simulink model "InvPendulum"  (R2018b)
settings: Solver=ode5  StartTime=0.0  StopTime=inf  FixedStep=0.01  RelTol=1e-3  AbsTol=1e-6
undefined symbols (not defined in the file): Standard_Devices, UDP_Protocol
libraries: sldrtlib x2, simulink x1
settings Model: ExtModeTrigDuration=18000  ExtModeTrigLevel=0.400000  Creator=jims  LastModifiedBy=Aleksei Tepljakov
settings SolverCC: AutoScaleAbsTol=off
settings DataIOCC: ExternalInput=[]  InitialState=[]  MaxDataPoints=5000  SaveFormat=Array  SignalLoggingSaveFormat=ModelDataLogs  SaveOutput=off  SaveTime=off
settings OptimizationCC: BooleanDataType=off  ExpressionDepthLimit=2147483647  LifeSpan=inf
settings DebuggingCC: SaveWithParameterizedLinksMsg=none  UnderspecifiedInitializationDetection=Classic  MergeDetectMultiDrivingBlocksExec=none  SignalResolutionControl=TryResolveAllWithWarning  MultiTaskDSMMsg=warning  MultiTaskCondExecSysMsg=none  IntegerOverflowMsg=none  FcnCallInpInsideContextMsg=warning  StateNameClashWarn=warning  SFUnexpectedBacktrackingDiag=warning  SFNoUnconditionalDefaultTransitionDiag=warning  SFExecutionAtInitializationDiag=none  IntegerSaturationMsg=none
settings HardwareCC: TargetBitPerLong=64  TargetBitPerPointer=64  TargetIntDivRoundTo=Zero  TargetEndianess=LittleEndian  TargetWordSize=64  TargetHWDeviceType=Intel->x86-64
settings ModelReferenceCC: PropagateSignalLabelsOutOfModel=off
settings SFSimCC: SimUseLocalCustomCode=off
settings RTWCC: SystemTargetFile=sldrt.tlc  TemplateMakefile=sldrt.tmf  Description=Simulink Desktop Real-Time  RTWUseLocalCustomCode=off  RTWCompilerOptimization=on
settings CodeAppCC: MaxIdLength=95  StateflowObjectComments=on
settings SimulinkDesktopRealTimeCC: TargetPreCompLibLocation=C:\Program Files\MATLAB\R2018b\toolbox\sldrt\lib\win64  TargetLangStandard=C89/C90 (ANSI)  SupportVariableSizeSignals=off  PreserveStateflowLocalDataDimensions=off
settings ConfigComp: CovMetricSettings=dw  CovHtmlReporting=on  CovSaveCumulativeToWorkspaceVar=on  CovSaveSingleToWorkspaceVar=on  CovExternalEMLEnable=off

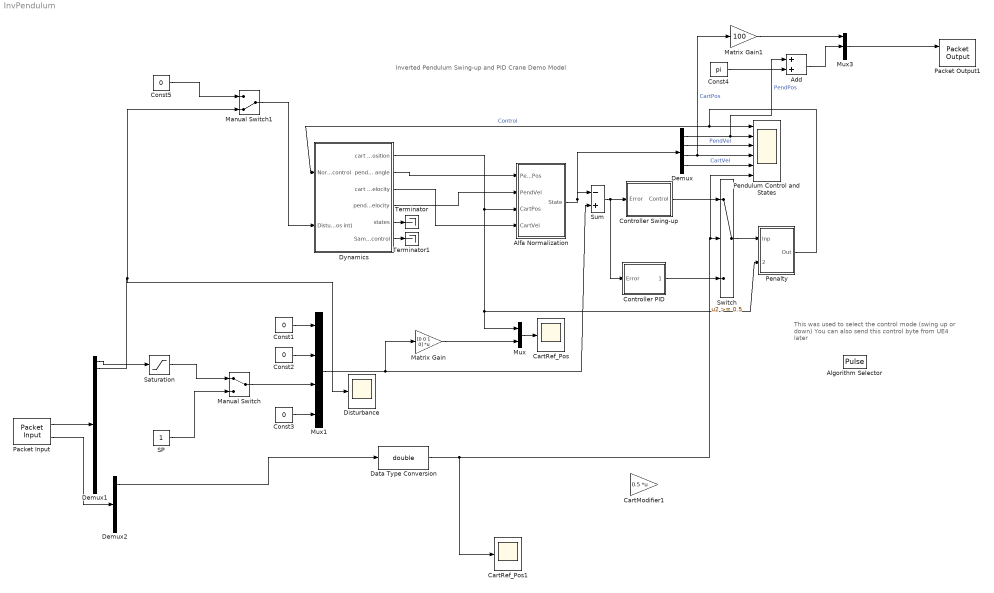
== system InvPendulum ==
  note: This was used to select
      | the control mode (swing up or down)
      | You can also send this control byte from UE4 later
  note: Inverted Pendulum
      | Swing-up and PID Crane Demo Model
  Add : Sum
  Alfa Normalization : Subsystem  mask(Choose mode:){}
  Algorithm Selector : DiscretePulseGenerator  PulseType=Time based  Period=30  PulseWidth=70
  CartModifier1 : Gain  Gain=0.5  Multiplication=Matrix(K*u)  SaturateOnIntegerOverflow=on  OutDataTypeStr=Inherit: Same as input  ParamDataTypeStr=Inherit: Same as input
  CartRef_Pos : Scope
  CartRef_Pos1 : Scope
  Const{1..3,5} (4 alike) : Constant  Value=0
  Const4 : Constant  Value=pi
  Controller PID : Subsystem  mask{Cart_PID=[ 0.5 0 0 ], Pend_PID=[ -1 0 -0.0 ], Umax=0.2, zone=1, Friction=0.03, T0=0.01}
      mask prompts: Cart_PID "Cart PID parameters [Kp, Ki, Kd]:"; Pend_PID "Pendulum PID parameters [Kp, Ki, Kd]:"; Umax "Maximum control value:"; zone "Stabilisation zone [rad]:"; Friction "Friction compensation:"; T0 "Sample time:"
  Controller Swing-up : Subsystem
  Data Type Conversion : DataTypeConversion  OutDataTypeStr=double
  Demux : Demux
  Demux1 : Demux  Outputs=20
  Demux2 : Demux  Outputs=3
  Disturbance : Scope
  Dynamics : Subsystem  mask(Dynamics){x_ini=[0, pi, 0, 0], m=[0.5723, 0.12], fr=[0.00027344,  1.1975875,  0.5], P4=[0.01955717, 0.0038583, 9.81], Up=[ 12.86, 0.093125], DZ=[0.1, 1.5]}
      mask prompts: x_ini "Initial state vector [x1(0)  x2(0)  x3(0)  x4(0)]"; m "mass of cart (mc)  mass of pendulum (mp)"; fr "friction :  fp  FS  FC"; P4 "Distance (l), Total Inertia moment (J), gravity (g)"; Up "control : magnitude (M)    DZu"; DZ "minimal velocities : cart (DZcv)  pendulum (DZcp)"
      mask help:
      | Pendulum-Cart Dynamics
      |
      | Copyright INTECO 1997
      mask init:
      | DZcv=DZ(1);DZcp=DZ(2);DZu=Up(2);l=P4(1);J=P4(2);g=P4(3);M=Up(1);mc=m(1);mp=m(2);fp=fr(1);FS=fr(2);FC=fr(3);mi=l*(mc+mp);a=l*l+J/(mc+mp);
      mask Display: plot(0,0,100,100,[40,48,48,40,40],[60,60,49,49,60],[37,44],[9,54],[100,8,4,1,0,100,100,0,40,100,100,0,0,40],[44,44,44,44,45,46,45,44,45,45,43,43,46,46],[100,48],[55,55],[0,40],[55,55])
  Manual Switch : ManualSwitch
  Manual Switch1 : ManualSwitch  CurrentSetting=0
  Matrix Gain : Gain  Gain=[0 0 1 0]  Multiplication=Matrix(K*u)  SaturateOnIntegerOverflow=on  OutDataTypeStr=Inherit: Same as input  ParamDataTypeStr=Inherit: Same as input
  Matrix Gain1 : Gain  Gain=100  SaturateOnIntegerOverflow=on  OutDataTypeStr=Inherit: Same as input  ParamDataTypeStr=Inherit: Same as input
  Mux : Mux  Inputs=2
  Mux1 : Mux
  Mux3 : Mux  Inputs=3
  Packet Input : sldrtlib/Packet Input  SampleTime=0.01  MaxMissedTicks=10  ShowMissedTicks=off  YieldWhenWaiting=off  DrvName=Standard_Devices/UDP_Protocol  DrvAddress=9977  DrvOptions=[0 16385 49 50 55 46 48 46 48 46 49 0 0 0 0 0 0 0 0 0 0 0 0 0 0 0 0 0 0 0 0 0 0 0 0 0 0 0 0 0 0 0 0 0 0 0 0 0 0 0 0 0 0 0 0 0 0 0 0 0 0 0 0 0 0 0 0 0 0 0 0 0 0 0 0 0 0 0 0 0 0 0 0 0 0 0 0 0 0 0 0 0 0 0 0 0 0 0 0 0 0 0 0 0 0 0 0 0 0 0 0 0 0 0 0 0 0 0 0 0 0 0 0 0 0 0 0 0 0 0 0 0 0 0 0 0 0 0 0 0 0 0 0 0 0 0 0 0 0 0 0 0 0 0 0 0 0 0 0 0 0 0 0 0 0 0 0 0 0 0 0 0 0 0 0 0 0 0 0 0 0 0 0 0 0 0 0 0 0 0 0 0 0 0 0 0 0 0 0 0 0 0 0 0 0 0 0 0 0 0 0 0 0 0 0 0 0 0 0 0 0 0 0 0 0 0 0 0 0 0 0 0 0 0 0 0 0 0 0 0 0 0 0 0 0 0 0 0 0 0 0 0 0 0 0 0]  PacketSize=83  DataTypes={'20*single', '3*uint8'}  ShowReady=off  ShowError=off  PacketID=1  ByteOrder=1  ShowTimestamp=off
      settings: AttributesFormatString=UDP Protocol [9977]  SourceProductName=Simulink Desktop Real-Time
  Packet Output1 : sldrtlib/Packet Output  SampleTime=0.01  MaxMissedTicks=25  ShowMissedTicks=on  YieldWhenWaiting=off  DrvName=Standard_Devices/UDP_Protocol  DrvAddress=9999  DrvOptions=[0 8888 49 50 55 46 48 46 48 46 49 0 0 0 0 0 0 0 0 0 0 0 0 0 0 0 0 0 0 0 0 0 0 0 0 0 0 0 0 0 0 0 0 0 0 0 0 0 0 0 0 0 0 0 0 0 0 0 0 0 0 0 0 0 0 0 0 0 0 0 0 0 0 0 0 0 0 0 0 0 0 0 0 0 0 0 0 0 0 0 0 0 0 0 0 0 0 0 0 0 0 0 0 0 0 0 0 0 0 0 0 0 0 0 0 0 0 0 0 0 0 0 0 0 0 0 0 0 0 0 0 0 0 0 0 0 0 0 0 0 0 0 0 0 0 0 0 0 0 0 0 0 0 0 0 0 0 0 0 0 0 0 0 0 0 0 0 0 0 0 0 0 0 0 0 0 0 0 0 0 0 0 0 0 0 0 0 0 0 0 0 0 0 0 0 0 0 0 0 0 0 0 0 0 0 0 0 0 0 0 0 0 0 0 0 0 0 0 0 0 0 0 0 0 0 0 0 0 0 0 0 0 0 0 0 0 0 0 0 0 0 0 0 0 0 0 0 0 0 0 0 0 0 0 0 0]  PacketSize=83  DataTypes={'20*single', '3*uint8'}  ShowReady=off  ShowError=off  PacketID=1  ByteOrder=1  InitialValue=[]  FinalValue=[]
      settings: AttributesFormatString=UDP Protocol [9999]  SourceProductName=Simulink Desktop Real-Time
  Penalty : Subsystem
  Pendulum Control and States : Scope  NumInputPorts=6
  "SP " : Constant
  Saturation : Saturate  UpperLimit=1.8  LowerLimit=0
  Sum : Sum  Inputs=|-+  SaturateOnIntegerOverflow=on  InputSameDT=on  OutDataTypeStr=Inherit: Same as first input
  Switch : Switch  Threshold=0.5  SaturateOnIntegerOverflow=on  InputSameDT=on
  Terminator : Terminator
  Terminator1 : Terminator
  wires:
  Sum/1 -> Controller PID/1(Error), Controller Swing-up/1(Error)
  Mux1/1 -> Matrix Gain/1, Sum/2
  Mux/1 -> CartRef_Pos/1
  Alfa Normalization/1(State) -> Demux/1, Sum/1
  Matrix Gain/1 -> Mux/2
  Penalty/1(Out) -> Dynamics/1(Normalized control), Pendulum Control and States/1  "Control"
  Controller Swing-up/1(Control) -> Switch/1
  Controller PID/1(Control) -> Switch/3
  Switch/1 -> Penalty/1(Inp)
  Demux/4 -> Pendulum Control and States/5  "CartVel"
  Demux/3 -> Matrix Gain1/1, Pendulum Control and States/4  "CartPos"
  Demux/2 -> Pendulum Control and States/3  "PendVel"
  Demux/1 -> Add/1, Pendulum Control and States/2  "PendPos"
  Dynamics/2(pendulum angle) -> Alfa Normalization/1(PendPos)
  Dynamics/4(pendulum velocity) -> Alfa Normalization/2(PendVel)
  Dynamics/1(cart position) -> Alfa Normalization/3(CartPos), Penalty/2(CartPos), Mux/1
  Dynamics/3(cart velocity) -> Alfa Normalization/4(CartVel)
  Dynamics/5(states) -> Terminator/1
  Dynamics/6(Sampled control) -> Terminator1/1
  Const3/1 -> Mux1/4
  Const2/1 -> Mux1/2
  Const1/1 -> Mux1/1
  Mux3/1 -> Packet Output1/1
  Manual Switch/1 -> Mux1/3
  Matrix Gain1/1 -> Mux3/1
  Const4/1 -> Add/2
  Add/1 -> Mux3/2
  Packet Input/1 -> Demux1/1
  Demux1/1 -> Saturation/1
  "SP "/1 -> Manual Switch/2
  Saturation/1 -> Manual Switch/1
  Data Type Conversion/1 -> CartRef_Pos1/1, Pendulum Control and States/6, Switch/2
  Packet Input/2 -> Demux2/1
  Demux2/1 -> Data Type Conversion/1
  Demux1/2 -> Manual Switch1/2, Disturbance/1
  Const5/1 -> Manual Switch1/1
  Manual Switch1/1 -> Dynamics/2(Disturb (to pos int))

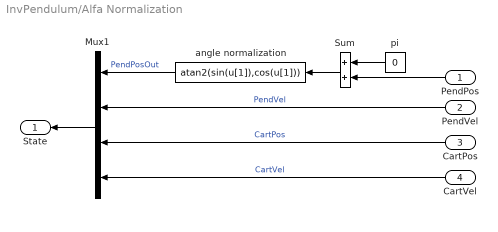
== system InvPendulum/Alfa Normalization ==
  PendPos : Inport
  PendVel : Inport  Port=2
  CartPos : Inport  Port=3
  CartVel : Inport  Port=4
  Mux1 : Mux
  Sum : Sum  SaturateOnIntegerOverflow=on  InputSameDT=on  OutDataTypeStr=Inherit: Same as first input
  angle normalization : Fcn  Expr=atan2(sin(u[1]),cos(u[1]))
  pi : Constant  Value=0
  State : Outport  InitialOutput=0
  wires:
  pi/1 -> Sum/1
  Sum/1 -> angle normalization/1
  Mux1/1 -> State/1
  CartPos/1 -> Mux1/3  "CartPos"
  CartVel/1 -> Mux1/4  "CartVel"
  PendVel/1 -> Mux1/2  "PendVel"
  PendPos/1 -> Sum/2
  angle normalization/1 -> Mux1/1  "PendPosOut"

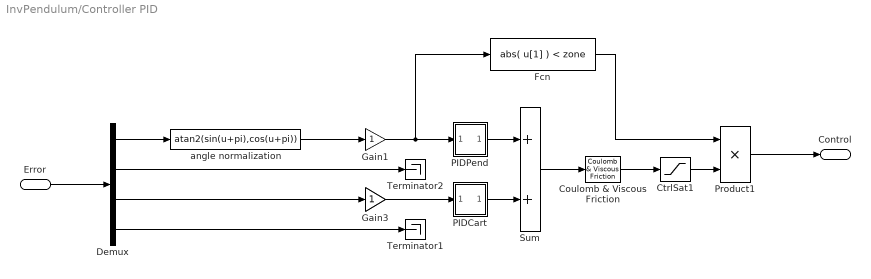
== system InvPendulum/Controller PID ==
  Error : Inport
  Coulomb & Viscous Friction : simulink/Discontinuities/Coulomb & Viscous Friction  offset=Friction  gain=1
      settings: SourceProductName=Simulink
  CtrlSat1 : Saturate  UpperLimit=Umax  LowerLimit=-Umax
  Demux : Demux
  Fcn : Fcn  Expr=abs( u[1] ) < zone
  Gain1 : Gain  SaturateOnIntegerOverflow=on  OutDataTypeStr=Inherit: Same as input  ParamDataTypeStr=Inherit: Same as input
  Gain3 : Gain  SaturateOnIntegerOverflow=on  OutDataTypeStr=Inherit: Same as input  ParamDataTypeStr=Inherit: Same as input
  PIDCart : Subsystem  mask(PID(2) Controller){P=Cart_PID(1), I=Cart_PID(2), D=Cart_PID(3), T0=T0}
      mask prompts: P "Proportional:"; I "Integral:"; D "Derivative:"; T0 "Sample Time:"
      mask help:
      | Enter Proportional(P), Integral(I), and Derivative(D) and divisor (N) terms.
      | P+I/s+Ds/(1/Ns+1)
      mask Help: This block implements a PID controller where parameters are entered for the Proportional, Integral and Derivative and divisor terms. Unmask this block to see how it works. The derivative term is implemented using an s/(s/N +1)  transfer function block. Making N large can create a "stiff" system.
      mask Display: disp('PID')
  PIDPend : Subsystem  mask(PID(2) Controller){P=Pend_PID(1), I=Pend_PID(2), D=Pend_PID(3), T0=T0}
      mask prompts: P "Proportional:"; I "Integral:"; D "Derivative:"; T0 "Sample Time:"
      mask help:
      | Enter Proportional(P), Integral(I), and Derivative(D) and divisor (N) terms.
      | P+I/s+Ds/(1/Ns+1)
      mask Help: This block implements a PID controller where parameters are entered for the Proportional, Integral and Derivative and divisor terms. Unmask this block to see how it works. The derivative term is implemented using an s/(s/N +1)  transfer function block. Making N large can create a "stiff" system.
      mask Display: disp('PID')
  Product1 : Product  SaturateOnIntegerOverflow=on  RndMeth=Zero  InputSameDT=on  OutDataTypeStr=Inherit: Same as first input
  Sum : Sum  SaturateOnIntegerOverflow=on  InputSameDT=on  OutDataTypeStr=Inherit: Same as first input
  Terminator1 : Terminator
  Terminator2 : Terminator
  angle normalization : Fcn  Expr=atan2(sin(u+pi),cos(u+pi))
  Control : Outport  InitialOutput=0
  wires:
  angle normalization/1 -> Gain1/1
  PIDCart/1(Out_1) -> Sum/2
  Gain3/1 -> PIDCart/1(In_1)
  Product1/1 -> Control/1
  Fcn/1 -> Product1/1
  CtrlSat1/1 -> Product1/2
  Coulomb & Viscous Friction/1 -> CtrlSat1/1
  Sum/1 -> Coulomb & Viscous Friction/1
  PIDPend/1(Out_1) -> Sum/1
  Gain1/1 -> PIDPend/1(In_1), Fcn/1
  Demux/1 -> angle normalization/1
  Error/1 -> Demux/1
  Demux/2 -> Terminator2/1
  Demux/3 -> Gain3/1
  Demux/4 -> Terminator1/1

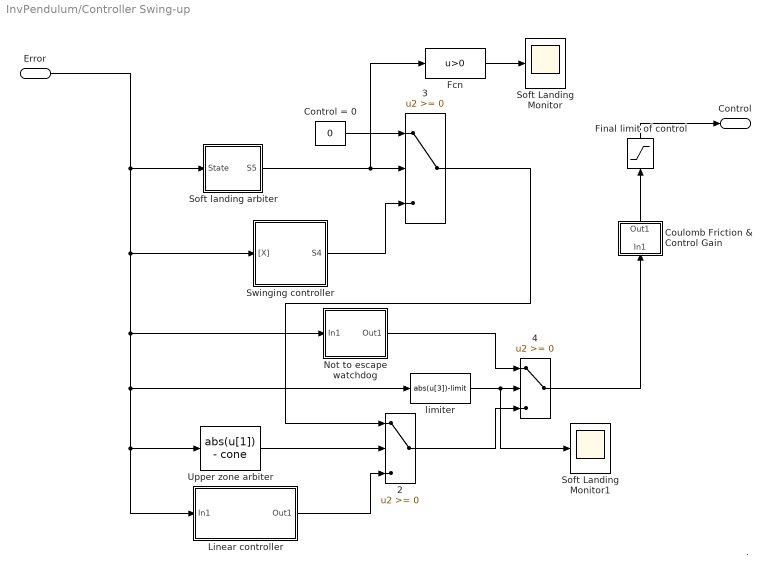
== system InvPendulum/Controller Swing-up ==
  note: .
  Error : Inport
  2 : Switch  SaturateOnIntegerOverflow=on  InputSameDT=on
  3 : Switch  SaturateOnIntegerOverflow=on  InputSameDT=on
  4 : Switch  SaturateOnIntegerOverflow=on  InputSameDT=on
  Control = 0 : Constant  Value=0
  Coulomb Friction & Control Gain : Subsystem  mask(Coulombic and Viscous Friction){friction=0.1, Umax=1}
      mask help:
      | A discontinuity offset at zero models coulomb friction.  Linear gain models viscous friction.
      | y = sign(x) * (Umax * abs(x) + friction)
      mask init:
      | x=max(friction(1),Umax(1)+friction(1));
      mask Help:
      | This block has a discontinuity
      | at zero and a linear gain afterward.
      | y= sign(x)*(Umax*abs(x)+friction)
      mask Display: plot([-1 0 0 1],[-friction(1)-Umax(1), -friction(1), friction(1), Umax(1)+friction(1)],[-1 1],[0 0],[0 0],[-x,x])
  Fcn : Fcn  Expr=u>0
  Final limit of control : Saturate  UpperLimit=0.2  LowerLimit=-0.2
  Linear controller : Subsystem  mask(linear){K4=-1.4, K2=0.6, K3=-0.8, K1=8.0}
      mask prompts: K4 "K4  - cart velocity feedback"; K2 "K2  - angle velocity feedback"; K3 "K3 - cart position feedback"; K1 "K1 - angle feedback"
      mask Display: plot(0,0,100,100,[40,30,20],[87,85,80],[46,54,54,46,46],[90,90,80,80,90],[46,45,45,46,54,55,55,54,46],[78,80,90,91,91,90,80,78,78],[51,51,49,49],[78,10,10,78],[90,80,70,60],[70,80,85,88],[20,10],[80,70],[20,20,15],[73,80,80],[85,80,80],[80,80,74])
  Not to escape watchdog : Subsystem  mask{umax2=1}
      mask prompts: umax2 "maximal force"
      mask Display: plot(0,0,100,100,[20,40,40,20,20],[60,60,49,49,60],[56,59,40],[58,55,55],[56,59],[52,55],[38,13,13],[39,39,46],[46,13],[46,46],[23,23,24,22,24,24,22,23],[47,45,49,48,48,46,47,49],[36,35,34,34,37,34,36,35,36,37,35,34,35],[49,48,46,49,48,47,45,47,48,46,46,47,49],[22,22,24,24],[46,49,48,47])
  Soft Landing Monitor : Scope
  Soft Landing Monitor1 : Scope
  Soft landing arbiter : Subsystem  mask(Soft landing){k=10.3, R=0.3}
      mask prompts: k "k coefficient"; R "R value"
      mask help: Soft landing
      mask Display: plot(0,0,100,100,[14,20,20,14,14],[20,20,8,8,20],[40,35,35,40,40],[39,40,51,51,40],[60,55,55,56,60,60],[70,70,60,60,60,71],[74,74,80,80,74],[80,91,91,80,80])
  Swinging controller : Subsystem  mask(swing){umax=1}
      mask prompts: umax "maximal control umax"
      mask help: swing
      mask Display: plot(0,0,100,100,[20,20],[12,87],[93,90,90,93,7],[50,46,54,50,50],[20,22,18,20],[87,80,80,88],[80,80,75,75,71,71,65,65,60,60,49,49,40,40,20],[50,40,40,60,60,50,50,80,80,20,21,80,80,21,20])
  Upper zone arbiter : Fcn  Expr=abs(u[1]) - cone  mask(ZONE){cone=0.3}
      mask prompts: cone "width of stabilization zone [rad]"
      mask help: ZONE
      mask Display: plot(0,0,100,100,[40,60,80,83,80,60,40,20,17,20,40],[89,89,80,70,60,51,51,60,69,80,90],[83,50,17],[70,8,68])
  limiter : Fcn  Expr=abs(u[3])-limit  mask{limit=0.35}
      mask prompts: limit "rail limit"
      mask Display: plot(0,0,100,100,[10,90,90,10],[52,52,50,50],[30,30],[52,60],[70,68,68,70,70],[60,60,52,52,60],[30,32,32,30],[52,52,60,60])
  Control : Outport  InitialOutput=0
  wires:
  Fcn/1 -> Soft Landing Monitor/1
  2/1 -> 4/3
  3/1 -> 2/1
  Swinging controller/1(S4) -> 3/3
  Control = 0/1 -> 3/1
  Soft landing arbiter/1(S5) -> Fcn/1, 3/2
  Error/1 -> Soft landing arbiter/1(State), Swinging controller/1("[X]"), limiter/1, Upper zone arbiter/1, Linear controller/1(In1), Not to escape watchdog/1(In1)
  limiter/1 -> 4/2, Soft Landing Monitor1/1
  Not to escape watchdog/1(Out1) -> 4/1
  Upper zone arbiter/1 -> 2/2
  Final limit of control/1 -> Control/1
  4/1 -> Coulomb Friction & Control Gain/1(In1)
  Linear controller/1(Out1) -> 2/3
  Coulomb Friction & Control Gain/1(Out1) -> Final limit of control/1

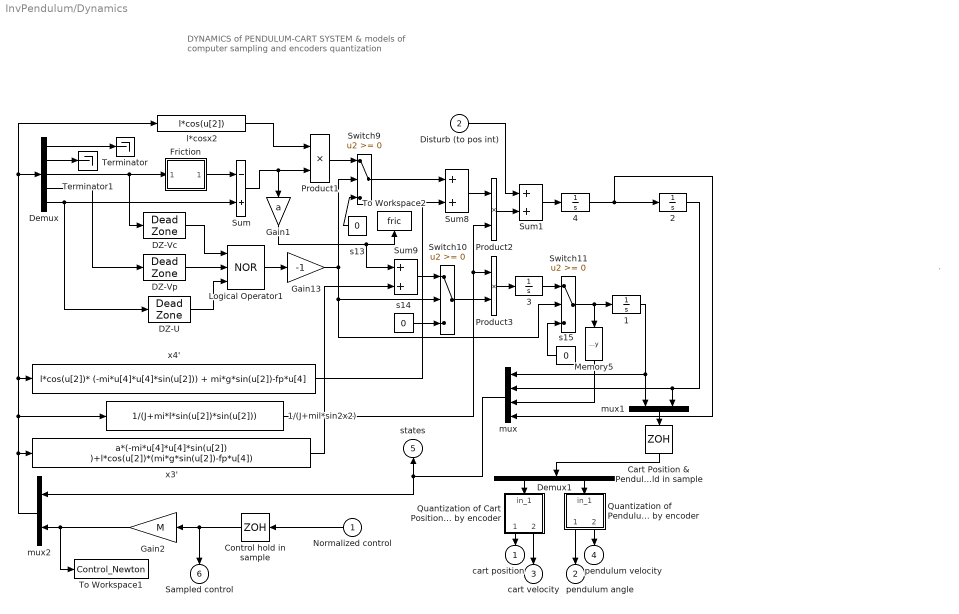
== system InvPendulum/Dynamics ==
  note: DYNAMICS of
      | PENDULUM-CART SYSTEM
      | & models of
      | computer sampling and encoders quantization
  note: .
  Normalized control : Inport
  Disturb (to pos int) : Inport  Port=2
  " Quantization of Pendulum Angle introduced by encoder" : Subsystem
  1 : Integrator  InitialCondition=x_ini(1)  LimitOutput=on  UpperSaturationLimit=1.9  LowerSaturationLimit=0
  1/(J+mil*sin2x2) : Fcn  Expr=1/(J+mi*l*sin(u[2])*sin(u[2]))
  2 : Integrator  InitialCondition=x_ini(2)
  3 : Integrator  InitialCondition=x_ini(3)
  4 : Integrator  InitialCondition=x_ini(4)
  Cart Position & Pendulum Angle hold in sample : ZeroOrderHold  SampleTime=0.01
  Control hold in sample : ZeroOrderHold  SampleTime=0.01
  DZ-U : DeadZone  LowerValue=-DZu  UpperValue=DZu  SaturateOnIntegerOverflow=on
  DZ-Vc : DeadZone  LowerValue=-DZcv  UpperValue=DZcv  SaturateOnIntegerOverflow=on
  DZ-Vp : DeadZone  LowerValue=-DZcp  UpperValue=DZcp  SaturateOnIntegerOverflow=on
  Demux : Demux  Outputs=5
  Demux1 : Demux  Outputs=2
  Friction : Subsystem  mask(Coulombic and Viscous Friction){FS=FS, FC=FC}
      mask prompts: FS "Static friction"; FC "Coulomb friction"
      mask help:
      | A discontinuity offset at zero models coulomb friction.  Linear gain models viscous friction.
      | y = sign(x) * (Umax * abs(x) + friction)
      mask Help:
      | This block has a discontinuity
      | at zero and a linear gain afterward.
      | y= sign(x)*(Umax*abs(x)+friction)
  Gain1 : Gain  Gain=a  SaturateOnIntegerOverflow=on  OutDataTypeStr=Inherit: Same as input  ParamDataTypeStr=Inherit: Same as input
  Gain13 : Gain  Gain=-1  SaturateOnIntegerOverflow=on  OutDataTypeStr=Inherit: Same as input  ParamDataTypeStr=Inherit: Same as input
  Gain2 : Gain  Gain=M  SaturateOnIntegerOverflow=on  OutDataTypeStr=Inherit: Same as input  ParamDataTypeStr=Inherit: Same as input
  Logical Operator1 : Logic  Operator=NOR  Inputs=3
  Memory5 : Memory
  Product1 : Product  SaturateOnIntegerOverflow=on  RndMeth=Zero  InputSameDT=on  OutDataTypeStr=Inherit: Same as first input
  Product2 : Product  SaturateOnIntegerOverflow=on  RndMeth=Zero  InputSameDT=on  OutDataTypeStr=Inherit: Same as first input
  Product3 : Product  SaturateOnIntegerOverflow=on  RndMeth=Zero  InputSameDT=on  OutDataTypeStr=Inherit: Same as first input
  "Quantization of Cart Position introduced by encoder " : Subsystem
  Sum : Sum  Inputs=-+  SaturateOnIntegerOverflow=on  InputSameDT=on  OutDataTypeStr=Inherit: Same as first input
  Sum1 : Sum  SaturateOnIntegerOverflow=on  InputSameDT=on  OutDataTypeStr=Inherit: Same as first input
  Sum8 : Sum  SaturateOnIntegerOverflow=on  InputSameDT=on  OutDataTypeStr=Inherit: Same as first input
  Sum9 : Sum  SaturateOnIntegerOverflow=on  InputSameDT=on  OutDataTypeStr=Inherit: Same as first input
  Switch10 : Switch  SaturateOnIntegerOverflow=on  InputSameDT=on
  Switch11 : Switch  SaturateOnIntegerOverflow=on  InputSameDT=on
  Switch9 : Switch  SaturateOnIntegerOverflow=on  InputSameDT=on
  Terminator : Terminator
  Terminator1 : Terminator
  To Workspace1 : ToWorkspace  VariableName=Control_Newton
      settings: MaxDataPoints=100000
  To Workspace2 : ToWorkspace  VariableName=fric
      settings: MaxDataPoints=100000
  l*cosx2 : Fcn  Expr=l*cos(u[2])
  mux : Mux
  mux1 : Mux  Inputs=2
  mux2 : Mux  Inputs=[4 1]
  s13 : Constant  Value=0
  s14 : Constant  Value=0
  s15 : Constant  Value=0
  x3' : Fcn  Expr=a*(-mi*u[4]*u[4]*sin(u[2]) )+l*cos(u[2])*(mi*g*sin(u[2])-fp*u[4])
  x4' : Fcn  Expr=l*cos(u[2])* (-mi*u[4]*u[4]*sin(u[2])) + mi*g*sin(u[2])-fp*u[4]
  cart position : Outport  InitialOutput=0
  pendulum angle : Outport  Port=2  InitialOutput=0
  cart velocity : Outport  Port=3  InitialOutput=0
  pendulum velocity : Outport  Port=4  InitialOutput=0
  states : Outport  Port=5  InitialOutput=0
  Sampled control : Outport  Port=6  InitialOutput=0
  wires:
  Demux1/1 -> "Quantization of Cart Position introduced by encoder "/1(in_1)
  mux/1 -> mux2/1, states/1
  "Quantization of Cart Position introduced by encoder "/1(out_1) -> cart position/1
  "Quantization of Cart Position introduced by encoder "/2(out_2) -> cart velocity/1
  " Quantization of Pendulum Angle introduced by encoder"/1(out_1) -> pendulum angle/1
  " Quantization of Pendulum Angle introduced by encoder"/2(out_2) -> pendulum velocity/1
  Demux1/2 -> " Quantization of Pendulum Angle introduced by encoder"/1(in_1)
  Control hold in sample/1 -> Sampled control/1, Gain2/1
  Normalized control/1 -> Control hold in sample/1
  Cart Position & Pendulum Angle hold in sample/1 -> Demux1/1
  mux1/1 -> Cart Position & Pendulum Angle hold in sample/1
  1/1 -> mux1/1, mux/1
  2/1 -> mux1/2, mux/2
  Switch11/1 -> Memory5/1, 1/1
  Memory5/1 -> mux/3
  Demux/2 -> Terminator1/1
  Demux/5 -> DZ-U/1, Sum/2
  Demux/1 -> Terminator/1
  Demux/4 -> DZ-Vp/1
  Demux/3 -> DZ-Vc/1, Friction/1(In1)
  DZ-U/1 -> Logical Operator1/3
  Logical Operator1/1 -> Gain13/1
  DZ-Vp/1 -> Logical Operator1/2
  DZ-Vc/1 -> Logical Operator1/1
  l*cosx2/1 -> Product1/1
  s13/1 -> Switch9/3
  Switch9/1 -> Sum8/1
  s14/1 -> Switch10/3
  Product1/1 -> Switch9/1
  x4'/1 -> Sum8/2
  Sum8/1 -> Product2/1
  Product2/1 -> Sum1/2
  Product3/1 -> 3/1
  Sum9/1 -> Switch10/1
  3/1 -> Switch11/1
  s15/1 -> Switch11/3
  Gain13/1 -> Switch9/2, Switch11/2, Switch10/2
  Switch10/1 -> Product3/2
  Sum/1 -> Product1/2, Gain1/1
  mux2/1 -> x3'/1, Demux/1, l*cosx2/1, x4'/1, 1/(J+mil*sin2x2)/1
  x3'/1 -> Sum9/2
  1/(J+mil*sin2x2)/1 -> Product2/2, Product3/1
  Gain1/1 -> Sum9/1, To Workspace2/1
  Gain2/1 -> To Workspace1/1, mux2/2
  Friction/1(Out1) -> Sum/1
  4/1 -> mux/4, 2/1
  Sum1/1 -> 4/1
  Disturb (to pos int)/1 -> Sum1/1

== system InvPendulum/Penalty ==
  Inp : Inport
  CartPos : Inport  Port=2
  CartRef_Pos1 : Scope
  CtrlSat : Saturate  UpperLimit=0.2  LowerLimit=-0.2
  Terminator1 : Terminator
  Out : Outport
  wires:
  CtrlSat/1 -> Out/1, CartRef_Pos1/1
  Inp/1 -> CtrlSat/1
  CartPos/1 -> Terminator1/1

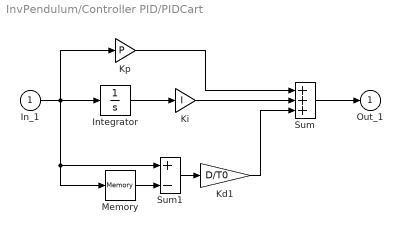
== system InvPendulum/Controller PID/PIDCart ==
  In_1 : Inport
  Integrator : Integrator  LimitOutput=on  UpperSaturationLimit=1  LowerSaturationLimit=-1
  Kd1 : Gain  Gain=D/T0  SaturateOnIntegerOverflow=on  OutDataTypeStr=Inherit: Same as input  ParamDataTypeStr=Inherit: Same as input
  Ki : Gain  Gain=I  SaturateOnIntegerOverflow=on  OutDataTypeStr=Inherit: Same as input  ParamDataTypeStr=Inherit: Same as input
  Kp : Gain  Gain=P  SaturateOnIntegerOverflow=on  OutDataTypeStr=Inherit: Same as input  ParamDataTypeStr=Inherit: Same as input
  Memory : Memory
  Sum : Sum  Inputs=+++  SaturateOnIntegerOverflow=on  InputSameDT=on  OutDataTypeStr=Inherit: Same as first input
  Sum1 : Sum  Inputs=+-  SaturateOnIntegerOverflow=on  InputSameDT=on  OutDataTypeStr=Inherit: Same as first input
  Out_1 : Outport  InitialOutput=0
  wires:
  Kd1/1 -> Sum/3
  Sum1/1 -> Kd1/1
  Memory/1 -> Sum1/2
  Kp/1 -> Sum/1
  Sum/1 -> Out_1/1
  In_1/1 -> Sum1/1, Memory/1, Kp/1, Integrator/1
  Integrator/1 -> Ki/1
  Ki/1 -> Sum/2

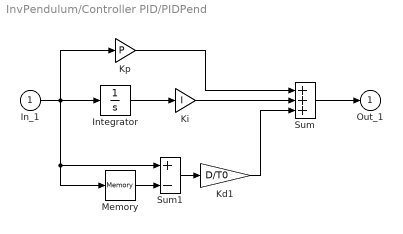
== system InvPendulum/Controller PID/PIDPend ==
  In_1 : Inport
  Integrator : Integrator  LimitOutput=on  UpperSaturationLimit=1  LowerSaturationLimit=-1
  Kd1 : Gain  Gain=D/T0  SaturateOnIntegerOverflow=on  OutDataTypeStr=Inherit: Same as input  ParamDataTypeStr=Inherit: Same as input
  Ki : Gain  Gain=I  SaturateOnIntegerOverflow=on  OutDataTypeStr=Inherit: Same as input  ParamDataTypeStr=Inherit: Same as input
  Kp : Gain  Gain=P  SaturateOnIntegerOverflow=on  OutDataTypeStr=Inherit: Same as input  ParamDataTypeStr=Inherit: Same as input
  Memory : Memory
  Sum : Sum  Inputs=+++  SaturateOnIntegerOverflow=on  InputSameDT=on  OutDataTypeStr=Inherit: Same as first input
  Sum1 : Sum  Inputs=+-  SaturateOnIntegerOverflow=on  InputSameDT=on  OutDataTypeStr=Inherit: Same as first input
  Out_1 : Outport  InitialOutput=0
  wires:
  Ki/1 -> Sum/2
  Integrator/1 -> Ki/1
  In_1/1 -> Integrator/1, Kp/1, Memory/1, Sum1/1
  Sum/1 -> Out_1/1
  Kp/1 -> Sum/1
  Memory/1 -> Sum1/2
  Sum1/1 -> Kd1/1
  Kd1/1 -> Sum/3

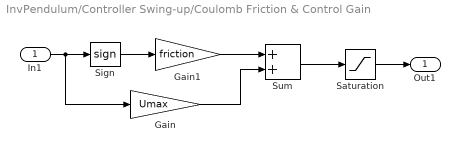
== system InvPendulum/Controller Swing-up/Coulomb Friction & Control Gain ==
  In1 : Inport
  Gain : Gain  Gain=Umax  SaturateOnIntegerOverflow=on  OutDataTypeStr=Inherit: Same as input  ParamDataTypeStr=Inherit: Same as input
  Gain1 : Gain  Gain=friction  SaturateOnIntegerOverflow=on  OutDataTypeStr=Inherit: Same as input  ParamDataTypeStr=Inherit: Same as input
  Saturation : Saturate  UpperLimit=1  LowerLimit=-1
  Sign : Signum
  Sum : Sum  SaturateOnIntegerOverflow=on  InputSameDT=on  OutDataTypeStr=Inherit: Same as first input
  Out1 : Outport  InitialOutput=0
  wires:
  Gain/1 -> Sum/2
  Gain1/1 -> Sum/1
  In1/1 -> Sign/1, Gain/1
  Sign/1 -> Gain1/1
  Sum/1 -> Saturation/1
  Saturation/1 -> Out1/1

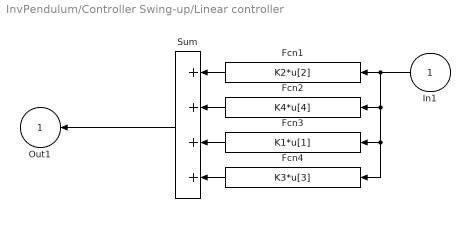
== system InvPendulum/Controller Swing-up/Linear controller ==
  In1 : Inport
  Fcn1 : Fcn  Expr=K2*u[2]
  Fcn2 : Fcn  Expr=K4*u[4]
  Fcn3 : Fcn  Expr=K1*u[1]
  Fcn4 : Fcn  Expr=K3*u[3]
  Sum : Sum  Inputs=++++  SaturateOnIntegerOverflow=on  InputSameDT=on  OutDataTypeStr=Inherit: Same as first input
  Out1 : Outport  InitialOutput=0
  wires:
  Sum/1 -> Out1/1
  Fcn2/1 -> Sum/2
  Fcn1/1 -> Sum/1
  In1/1 -> Fcn1/1, Fcn2/1, Fcn3/1, Fcn4/1
  Fcn3/1 -> Sum/3
  Fcn4/1 -> Sum/4

== system InvPendulum/Controller Swing-up/Not to escape watchdog ==
  In1 : Inport
  Fcn : Fcn  Expr=u[3]
  Gain : Gain  Gain=umax2  SaturateOnIntegerOverflow=on  OutDataTypeStr=Inherit: Same as input  ParamDataTypeStr=Inherit: Same as input
  Sign : Signum
  Out1 : Outport  InitialOutput=0
  wires:
  Sign/1 -> Gain/1
  Gain/1 -> Out1/1
  Fcn/1 -> Sign/1
  In1/1 -> Fcn/1

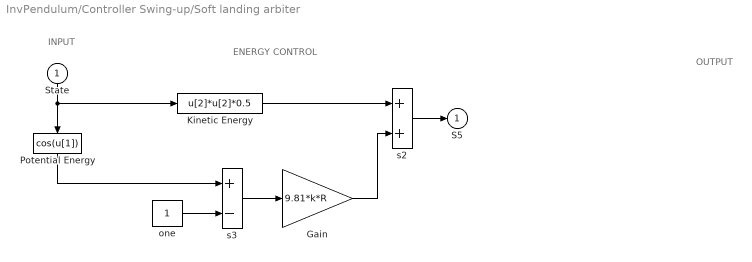
== system InvPendulum/Controller Swing-up/Soft landing arbiter ==
  note: ENERGY CONTROL
  note: OUTPUT
  note: INPUT
  State : Inport
  Gain : Gain  Gain=9.81*k*R  SaturateOnIntegerOverflow=on  OutDataTypeStr=Inherit: Same as input  ParamDataTypeStr=Inherit: Same as input
  Kinetic Energy : Fcn  Expr=u[2]*u[2]*0.5
  Potential Energy : Fcn  Expr=cos(u[1])
  "one " : Constant
  s2 : Sum  SaturateOnIntegerOverflow=on  InputSameDT=on  OutDataTypeStr=Inherit: Same as first input
  s3 : Sum  Inputs=+-  SaturateOnIntegerOverflow=on  InputSameDT=on  OutDataTypeStr=Inherit: Same as first input
  S5 : Outport  InitialOutput=0
  wires:
  Potential Energy/1 -> s3/1
  "one "/1 -> s3/2
  Kinetic Energy/1 -> s2/1
  s3/1 -> Gain/1
  Gain/1 -> s2/2
  State/1 -> Potential Energy/1, Kinetic Energy/1
  s2/1 -> S5/1

== system InvPendulum/Controller Swing-up/Swinging controller ==
  "[X]" : Inport
  Saturation : Saturate  UpperLimit=umax  LowerLimit=-umax
  abs(x1) : Fcn  Expr=u[2]*(abs(u[1])-pi/2)
  swing : Relay  OffOutputValue=-1
  umax : Gain  Gain=umax  SaturateOnIntegerOverflow=on  OutDataTypeStr=Inherit: Same as input  ParamDataTypeStr=Inherit: Same as input
  S4 : Outport  InitialOutput=0
  wires:
  umax/1 -> Saturation/1
  "[X]"/1 -> abs(x1)/1
  swing/1 -> umax/1
  abs(x1)/1 -> swing/1
  Saturation/1 -> S4/1

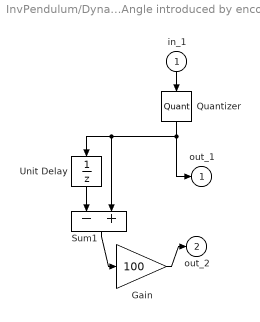
== system InvPendulum/Dynamics/ Quantization of Pendulum Angle introduced by encoder ==
  in_1 : Inport
  Gain : Gain  Gain=100  SaturateOnIntegerOverflow=on  OutDataTypeStr=Inherit: Same as input  ParamDataTypeStr=Inherit: Same as input
  Quantizer : Quantizer  QuantizationInterval=0.001534
  Sum1 : Sum  Inputs=-+  SaturateOnIntegerOverflow=on  InputSameDT=on  OutDataTypeStr=Inherit: Same as first input
  Unit Delay : UnitDelay  InitialCondition=x_ini(2)  SampleTime=0.01
  out_1 : Outport  InitialOutput=0
  out_2 : Outport  Port=2  InitialOutput=0
  wires:
  in_1/1 -> Quantizer/1
  Quantizer/1 -> Sum1/2, Unit Delay/1, out_1/1
  Sum1/1 -> Gain/1
  Gain/1 -> out_2/1
  Unit Delay/1 -> Sum1/1

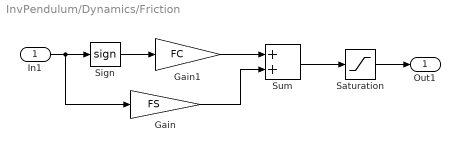
== system InvPendulum/Dynamics/Friction ==
  In1 : Inport
  Gain : Gain  Gain=FS  SaturateOnIntegerOverflow=on  OutDataTypeStr=Inherit: Same as input  ParamDataTypeStr=Inherit: Same as input
  Gain1 : Gain  Gain=FC  SaturateOnIntegerOverflow=on  OutDataTypeStr=Inherit: Same as input  ParamDataTypeStr=Inherit: Same as input
  Saturation : Saturate  UpperLimit=1  LowerLimit=-1
  Sign : Signum
  Sum : Sum  SaturateOnIntegerOverflow=on  InputSameDT=on  OutDataTypeStr=Inherit: Same as first input
  Out1 : Outport  InitialOutput=0
  wires:
  Saturation/1 -> Out1/1
  Sum/1 -> Saturation/1
  Sign/1 -> Gain1/1
  In1/1 -> Gain/1, Sign/1
  Gain1/1 -> Sum/1
  Gain/1 -> Sum/2

== system InvPendulum/Dynamics/Quantization of Cart Position introduced by encoder  ==
  in_1 : Inport
  Gain : Gain  Gain=100  SaturateOnIntegerOverflow=on  OutDataTypeStr=Inherit: Same as input  ParamDataTypeStr=Inherit: Same as input
  Quantizer1 : Quantizer  QuantizationInterval=5.7053e-005
  Sum1 : Sum  Inputs=-+  SaturateOnIntegerOverflow=on  InputSameDT=on  OutDataTypeStr=Inherit: Same as first input
  Unit Delay : UnitDelay  InitialCondition=x_ini(1)  SampleTime=0.01
  out_1 : Outport  InitialOutput=0
  out_2 : Outport  Port=2  InitialOutput=0
  wires:
  Quantizer1/1 -> Sum1/2, Unit Delay/1, out_1/1
  Unit Delay/1 -> Sum1/1
  Gain/1 -> out_2/1
  in_1/1 -> Quantizer1/1
  Sum1/1 -> Gain/1
